simulink model "untitled1"  (R2022b)
settings: Solver=FixedStepDiscrete  StartTime=0.0  StopTime=inf  FixedStep=1e-3  RelTol=1e-3  EnableMultiTasking=on
libraries: arduinolib x5
settings Model: ExtModeTrigDuration=2  Creator=yasso  LastModifiedBy=yasso
settings OptimizationCC: EnhancedBackFolding=on  PassReuseOutputArgsAs=Individual arguments  ZeroExternalMemoryAtStartup=off  ZeroInternalMemoryAtStartup=off  MaxStackSize=64  OptimizeBlockOrder=speed  DifferentSizesBufferReuse=on  OptimizationCustomize=off  EfficientTunableParamExpr=on
settings DebuggingCC: ParameterTunabilityLossMsg=error
settings HardwareCC: ProdBitPerInt=16  ProdBitPerPointer=16  ProdBitPerSizeT=16  ProdBitPerPtrDiffT=16  ProdLargestAtomicFloat=None  ProdWordSize=8  ProdHWDeviceType=Atmel->AVR
settings SFSimCC: MATLABDynamicMemAlloc=off
settings RTWCC: Description=Embedded Coder  SystemTargetFile=ert.tlc  HardwareBoard=Arduino Uno  TLCOptions=-aInlineSetEventsForThisBaseRateFcn=TLC_FALSE -aSuppressMultiTaskScheduler=TLC_FALSE -aRateBasedStepFcn=1  TemplateMakefile=ert_default_tmf  Toolchain=Arduino AVR  BuildConfiguration=Faster Runs
settings CodeAppCC: ForceParamTrailComments=on  IgnoreCustomStorageClasses=off  OperatorAnnotations=on  SimulinkDataObjDesc=on  SFDataObjDesc=on  InsertBlockDesc=on
settings ERTTargetCC: SupportContinuousTime=on  SupportVariableSizeSignals=on  ExtModeTransport=3  ExtModeStaticAlloc=on  ExtModeAutomaticAllocSize=off  ExtModeStaticAllocSize=250  ExtModeMexFile=ext_xcp  ExtModeIntrfLevel=Level2 - Open

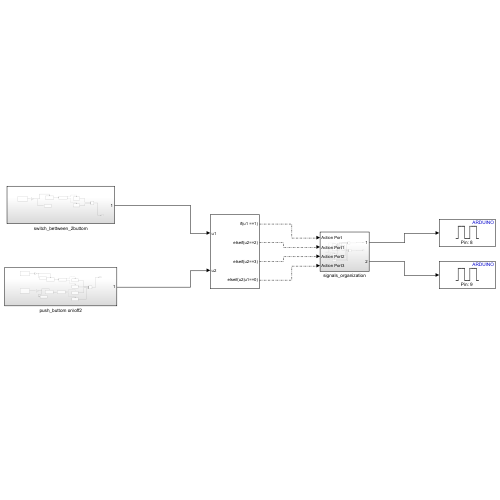
[thumbnail: Simulink's stored preview of the top-level diagram]
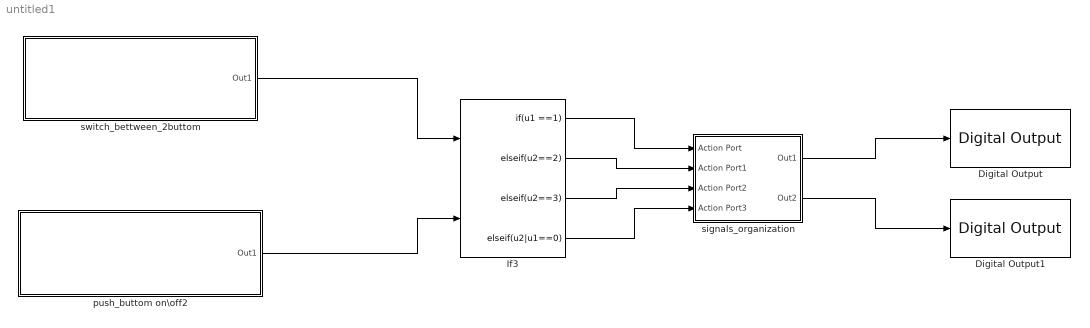
== system untitled1 ==
  Digital Output : arduinolib/Digital Output  pinNumber=8  Direction=output  blockPlatform=arduino
  Digital Output1 : arduinolib/Digital Output  pinNumber=9  Direction=output  blockPlatform=arduino
  If3 : If  NumInputs=2  IfExpression=u1 ==1  ElseIfExpressions=u2==2,u2==3,u2|u1==0  ShowElse=off
  push_buttom on\off2 : Subsystem
  signals_organization : Subsystem
  switch_bettween_2buttom : Subsystem
  wires:
  switch_bettween_2buttom/1(Out1) -> If3/1
  signals_organization/1(Out1) -> Digital Output/1
  If3/2 -> signals_organization/2(Action Port1)
  If3/1 -> signals_organization/1(Action Port)
  signals_organization/2(Out2) -> Digital Output1/1
  If3/3 -> signals_organization/3(Action Port2)
  push_buttom on\off2/1(Out1) -> If3/2
  If3/4 -> signals_organization/4(Action Port3)

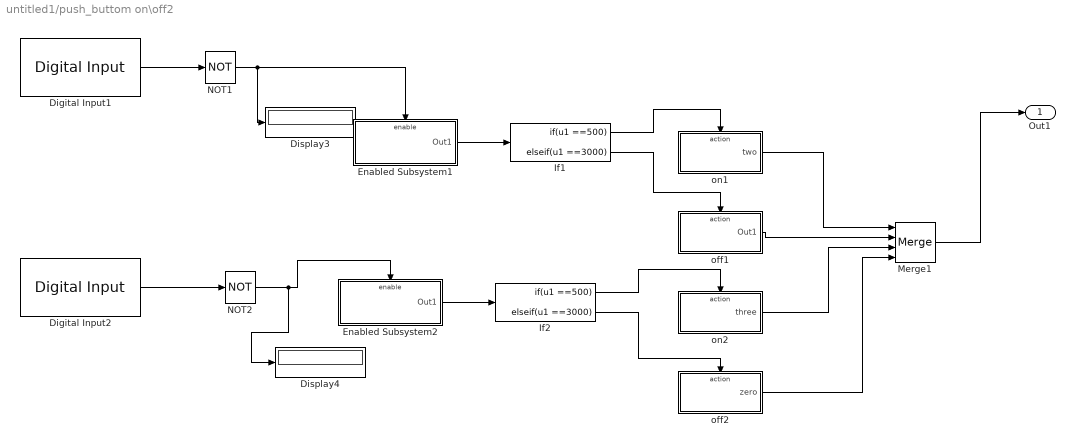
== system untitled1/push_buttom on\off2 ==
  Digital Input1 : arduinolib/Digital Input  pinNumber=4  mode=Input Pullup  Direction=input  SampleTime=1e-3  blockPlatform=arduino
  Digital Input2 : arduinolib/Digital Input  pinNumber=7  mode=Input Pullup  Direction=input  SampleTime=1e-3  blockPlatform=arduino
  Display3 : Display
  Display4 : Display
  Enabled Subsystem1 : Subsystem  TreatAsAtomicUnit=on
  Enabled Subsystem2 : Subsystem  TreatAsAtomicUnit=on
  If1 : If  IfExpression=u1 ==500  ElseIfExpressions=u1 ==3000  ShowElse=off
  If2 : If  IfExpression=u1 ==500  ElseIfExpressions=u1 ==3000  ShowElse=off
  Merge1 : Merge  Inputs=4
  NOT1 : Logic  Operator=NOT  IconShape=distinctive  AllPortsSameDT=off  OutDataTypeStr=boolean
  NOT2 : Logic  Operator=NOT  IconShape=distinctive  AllPortsSameDT=off  OutDataTypeStr=boolean
  off1 : Subsystem  TreatAsAtomicUnit=on
  off2 : Subsystem  TreatAsAtomicUnit=on
  on1 : Subsystem  TreatAsAtomicUnit=on
  on2 : Subsystem  TreatAsAtomicUnit=on
  Out1 : Outport
  wires:
  If2/1 -> on2/Action
  If1/2 -> off1/Action
  NOT2/1 -> Display4/1, Enabled Subsystem2/Enable
  Digital Input1/1 -> NOT1/1
  Enabled Subsystem1/1(Out1) -> If1/1
  If2/2 -> off2/Action
  off1/1(Out1) -> Merge1/2
  off2/1(zero) -> Merge1/4
  NOT1/1 -> Display3/1, Enabled Subsystem1/Enable
  Enabled Subsystem2/1(Out1) -> If2/1
  If1/1 -> on1/Action
  on1/1(two) -> Merge1/1
  on2/1(three) -> Merge1/3
  Digital Input2/1 -> NOT2/1
  Merge1/1 -> Out1/1

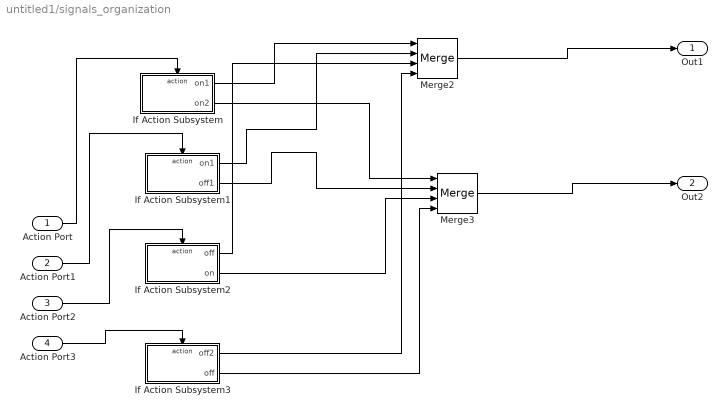
== system untitled1/signals_organization ==
  Action Port : Inport
  Action Port1 : Inport  Port=2
  Action Port2 : Inport  Port=3
  Action Port3 : Inport  Port=4
  If Action Subsystem : Subsystem  TreatAsAtomicUnit=on
  If Action Subsystem1 : Subsystem  TreatAsAtomicUnit=on
  If Action Subsystem2 : Subsystem  TreatAsAtomicUnit=on
  If Action Subsystem3 : Subsystem  TreatAsAtomicUnit=on
  Merge2 : Merge  Inputs=4
  Merge3 : Merge  Inputs=4
  Out1 : Outport
  Out2 : Outport  Port=2
  wires:
  Action Port3/1 -> If Action Subsystem3/Action
  If Action Subsystem/2(on2) -> Merge3/1
  If Action Subsystem3/2(off) -> Merge3/4
  If Action Subsystem1/2(off1) -> Merge3/2
  If Action Subsystem1/1(on1) -> Merge2/2
  If Action Subsystem2/1(off) -> Merge2/3
  Action Port1/1 -> If Action Subsystem1/Action
  If Action Subsystem2/2(on) -> Merge3/3
  Merge3/1 -> Out2/1
  If Action Subsystem3/1(off2) -> Merge2/4
  If Action Subsystem/1(on1) -> Merge2/1
  Action Port2/1 -> If Action Subsystem2/Action
  Action Port/1 -> If Action Subsystem/Action
  Merge2/1 -> Out1/1

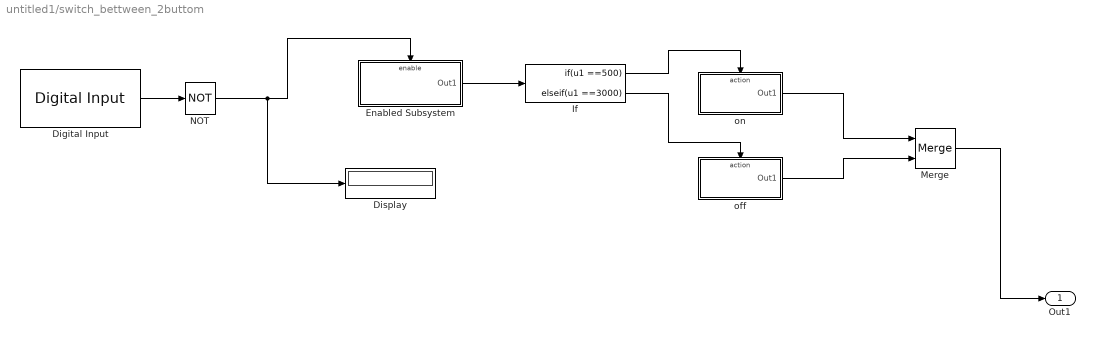
== system untitled1/switch_bettween_2buttom ==
  Digital Input : arduinolib/Digital Input  pinNumber=2  mode=Input Pullup  Direction=input  SampleTime=1e-3  blockPlatform=arduino
  Display : Display
  Enabled Subsystem : Subsystem  TreatAsAtomicUnit=on
  If : If  IfExpression=u1 ==500  ElseIfExpressions=u1 ==3000  ShowElse=off
  Merge : Merge
  NOT : Logic  Operator=NOT  IconShape=distinctive  AllPortsSameDT=off  OutDataTypeStr=boolean
  off : Subsystem  TreatAsAtomicUnit=on
  on : Subsystem  TreatAsAtomicUnit=on
  Out1 : Outport
  wires:
  If/2 -> off/Action
  Digital Input/1 -> NOT/1
  If/1 -> on/Action
  Enabled Subsystem/1(Out1) -> If/1
  on/1(Out1) -> Merge/1
  NOT/1 -> Display/1, Enabled Subsystem/Enable
  off/1(Out1) -> Merge/2
  Merge/1 -> Out1/1

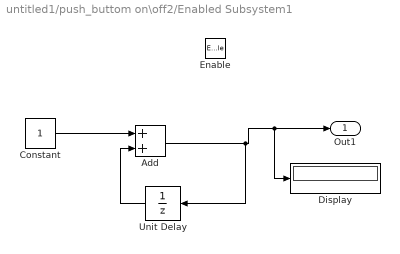
== system untitled1/push_buttom on\off2/Enabled Subsystem1 ==
  Enable : EnablePort  StatesWhenEnabling=reset
  Add : Sum
  Constant : Constant
  Display : Display
  Unit Delay : UnitDelay  SampleTime=-1  HasFrameUpgradeWarning=on
  Out1 : Outport
  wires:
  Unit Delay/1 -> Add/2
  Add/1 -> Display/1, Out1/1, Unit Delay/1
  Constant/1 -> Add/1

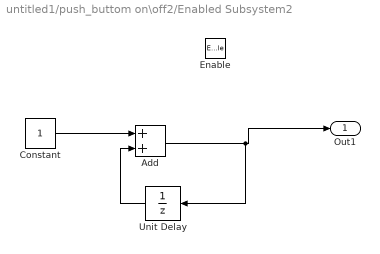
== system untitled1/push_buttom on\off2/Enabled Subsystem2 ==
  Enable : EnablePort  StatesWhenEnabling=reset
  Add : Sum
  Constant : Constant
  Unit Delay : UnitDelay  SampleTime=-1  HasFrameUpgradeWarning=on
  Out1 : Outport
  wires:
  Constant/1 -> Add/1
  Add/1 -> Unit Delay/1, Out1/1
  Unit Delay/1 -> Add/2

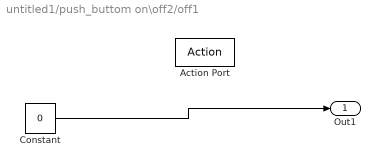
== system untitled1/push_buttom on\off2/off1 ==
  Action Port : ActionPort  ActionPortLabel=elseif(u1 ==3000)
  Constant : Constant  Value=0
  Out1 : Outport
  wires:
  Constant/1 -> Out1/1

== system untitled1/push_buttom on\off2/off2 ==
  Action Port : ActionPort  ActionPortLabel=elseif(u1 ==3000)
  Constant : Constant  Value=0
  zero : Outport
  wires:
  Constant/1 -> zero/1

== system untitled1/push_buttom on\off2/on1 ==
  Action Port : ActionPort  ActionPortLabel=if(u1 ==500)
  Constant : Constant  Value=2
  two : Outport
  wires:
  Constant/1 -> two/1

== system untitled1/push_buttom on\off2/on2 ==
  Action Port : ActionPort  ActionPortLabel=if(u1 ==500)
  Constant : Constant  Value=3
  three : Outport
  wires:
  Constant/1 -> three/1

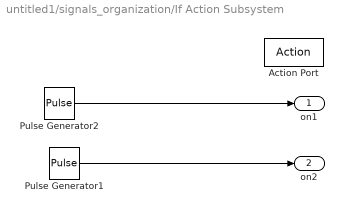
== system untitled1/signals_organization/If Action Subsystem ==
  Action Port : ActionPort  ActionPortLabel=if(u1 ==1)
  Pulse Generator1 : DiscretePulseGenerator  PulseType=Time based  Period=1  PulseWidth=50
  Pulse Generator2 : DiscretePulseGenerator  PulseType=Time based  Period=1  PulseWidth=50
  on1 : Outport
  on2 : Outport  Port=2
  wires:
  Pulse Generator2/1 -> on1/1
  Pulse Generator1/1 -> on2/1

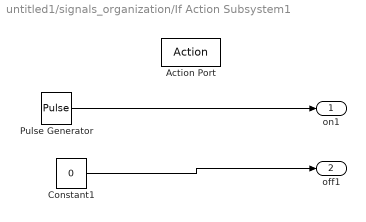
== system untitled1/signals_organization/If Action Subsystem1 ==
  Action Port : ActionPort  ActionPortLabel=elseif(u2==2)
  Constant1 : Constant  Value=0
  Pulse Generator : DiscretePulseGenerator  PulseType=Time based  PulseWidth=50
  on1 : Outport
  off1 : Outport  Port=2
  wires:
  Constant1/1 -> off1/1
  Pulse Generator/1 -> on1/1

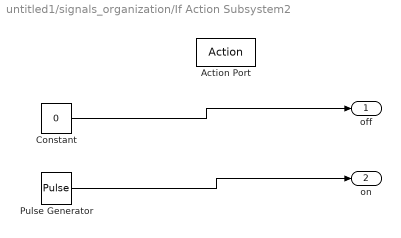
== system untitled1/signals_organization/If Action Subsystem2 ==
  Action Port : ActionPort  ActionPortLabel=elseif(u2==3)
  Constant : Constant  Value=0
  Pulse Generator : DiscretePulseGenerator  PulseType=Time based  PulseWidth=50
  off : Outport
  on : Outport  Port=2
  wires:
  Constant/1 -> off/1
  Pulse Generator/1 -> on/1

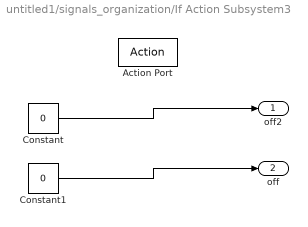
== system untitled1/signals_organization/If Action Subsystem3 ==
  Action Port : ActionPort  ActionPortLabel=elseif(u2|u1==0)
  Constant : Constant  Value=0
  Constant1 : Constant  Value=0
  off2 : Outport
  off : Outport  Port=2
  wires:
  Constant/1 -> off2/1
  Constant1/1 -> off/1

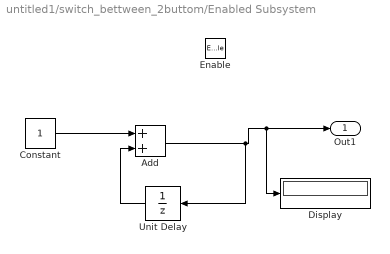
== system untitled1/switch_bettween_2buttom/Enabled Subsystem ==
  Enable : EnablePort  StatesWhenEnabling=reset
  Add : Sum
  Constant : Constant
  Display : Display
  Unit Delay : UnitDelay  SampleTime=-1  HasFrameUpgradeWarning=on
  Out1 : Outport
  wires:
  Constant/1 -> Add/1
  Add/1 -> Unit Delay/1, Display/1, Out1/1
  Unit Delay/1 -> Add/2

== system untitled1/switch_bettween_2buttom/off ==
  Action Port : ActionPort  ActionPortLabel=elseif(u1 ==3000)
  Constant : Constant  Value=0
  Out1 : Outport
  wires:
  Constant/1 -> Out1/1

== system untitled1/switch_bettween_2buttom/on ==
  Action Port : ActionPort  ActionPortLabel=if(u1 ==500)
  Constant : Constant
  Out1 : Outport
  wires:
  Constant/1 -> Out1/1
